simulink model "Task_3"  (R2017b)
settings: Solver=VariableStepAuto  StartTime=0.0  StopTime=0.05  RelTol=1e-3
settings Model: Creator=Ruslan  LastModifiedBy=Ruslan

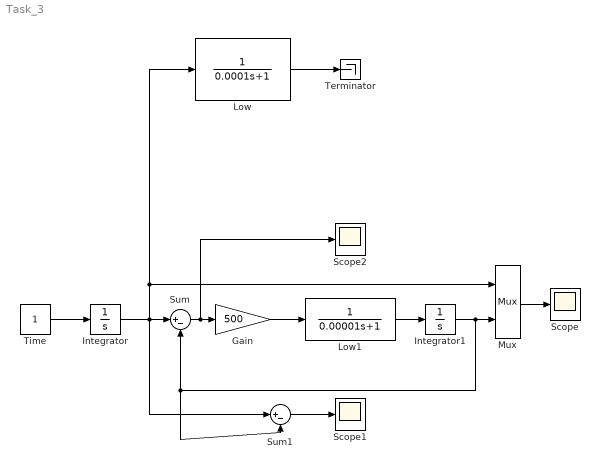
== system Task_3 ==
  Gain : Gain  Gain=500
  Integrator : Integrator
  Integrator1 : Integrator
  Low : TransferFcn  Denominator=[0.0001 1]
  Low1 : TransferFcn  Denominator=[0.00001 1]
  Mux : Mux  Inputs=2
  Scope : Scope
  Scope1 : Scope
  Scope2 : Scope
  Sum : Sum  Inputs=|+-
  Sum1 : Sum  Inputs=|+-
  Terminator : Terminator
  Time : Constant
  wires:
  Time/1 -> Integrator/1
  Low/1 -> Terminator/1
  Integrator/1 -> Sum1/1, Low/1, Mux/1, Sum/1
  Sum/1 -> Scope2/1, Gain/1
  Gain/1 -> Low1/1
  Low1/1 -> Integrator1/1
  Integrator1/1 -> Mux/2, Sum1/2, Sum/2
  Mux/1 -> Scope/1
  Sum1/1 -> Scope1/1
